simulink model "QCar_Workspace_studio"  (R2022b)
settings: Solver=ode1  StartTime=0.0  StopTime=inf  FixedStep=1/500  RelTol=1e-3  EnableMultiTasking=on
model workspace (MAT data in the model file):
  cameraStepSize = Simulink.Parameter
  cameraStepSize.Value = Simulink.data.Expression
  cameraStepSize.Value.ExpressionString = "qc_get_step_size * 2 + 0*ceil (1/90 /qc_get_step_size)"
  cameraStepSize.DataType = 'auto'
  cameraStepSize.Complexity = 'real'
  cameraStepSize.Dimensions = -1
  internalStepSize = Simulink.Parameter
  internalStepSize.Value = Simulink.data.Expression
  internalStepSize.Value.ExpressionString = "qc_get_step_size * ceil(1/120 /qc_get_step_size)"
  internalStepSize.DataType = 'auto'
  internalStepSize.Complexity = 'real'
  internalStepSize.Dimensions = -1
  mainStepSize = Simulink.Parameter
  mainStepSize.Value = Simulink.data.Expression
  mainStepSize.Value.ExpressionString = "qc_get_step_size"
  mainStepSize.DataType = 'auto'
  mainStepSize.Complexity = 'real'
  mainStepSize.Dimensions = -1
undefined symbols (not defined in the file or in its folder): qc_get_step_size
libraries: quarc_library x44, simulink x5
(part 1 of 2)
settings Model: SimulationMode=external  ExtModeTrigDuration=10000  Creator=mbohra  LastModifiedBy=mbohra
settings SolverCC: AlgebraicLoopSolver=TrustRegion  PositivePriorityOrder=on
settings DataIOCC: SaveOutput=off  SignalLogging=off  DSMLogging=off  SaveTime=off  ReturnWorkspaceOutputs=off
settings DebuggingCC: UnconnectedInputMsg=warning  UnconnectedOutputMsg=warning  UnconnectedLineMsg=warning  SFMachineParentedDataDiag=warning  ArithmeticOperatorsInVariantConditions=warning
settings ModelReferenceCC: EnableRefExpFcnMdlSchedulingChecks=on
settings SFSimCC: SimUseLocalCustomCode=off  CustomCodeUndefinedFunction=UseInterfaceOnly
settings RTWCC: Description=QUARC Win64 Target Using Toolchain  SystemTargetFile=quarc_win64.tlc  TemplateMakefile=quarc_default_tmf  RTWUseLocalCustomCode=off  Toolchain=QUARC win64 | nmake (64-bit Windows)  BuildConfiguration=Faster Runs  DLArmComputeVersion=19.05
settings CodeAppCC: StateflowObjectComments=on
settings STFCustomTargetCC: TargetLangStandard=C99 (ISO)  ConcurrentExecutionCompliant=on  GRTInterface=on  UseToolchainInfoCompliant=on  SystemTargetFile=quarc_win64.tlc
settings GRTTargetCC: ParMdlRefBuildCompliant=off  CompOptLevelCompliant=off  CombineOutputUpdateFcns=off  MatFileLogging=off  CPPClassGenCompliant=off  GRTInterface=on  ExtMode=on  ExtModeMexFile=quarc_comm
settings ConfigComp: CovMetricSettings=dswe

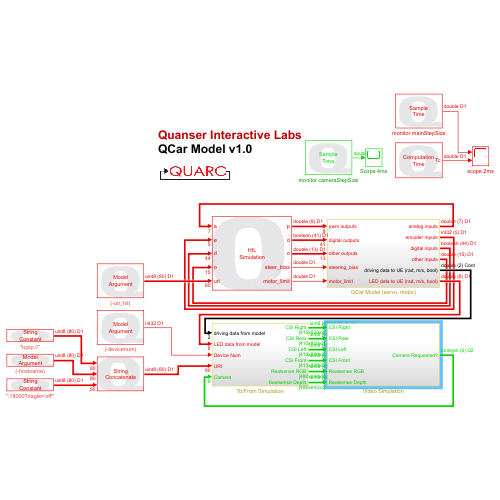
[thumbnail: Simulink's stored preview of the top-level diagram]
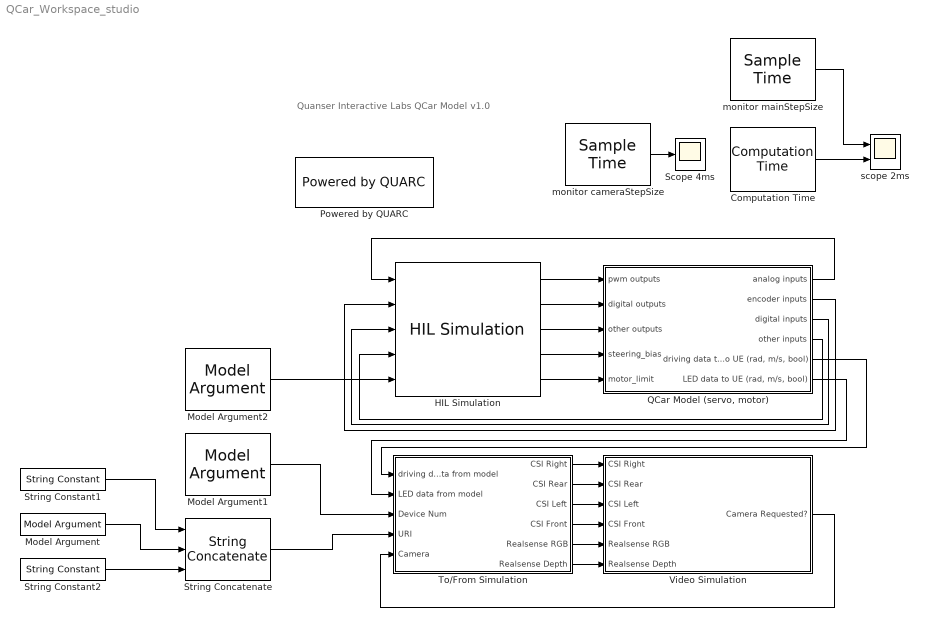
== system QCar_Workspace_studio ==
  note: Quanser Interactive Labs
      | QCar Model v1.0
  Computation Time : quarc_library/Sources/Time/Computation Time  sample_time=mainStepSize  use_model=on  use_cpu_time=off
  HIL Simulation : quarc_library/Data Acquisition/Generic/Configuration/HIL Simulation  uri_source=External input port  uri=tcpip://localhost:18960  board_type=qcar  board_id=0  options=steer_bias=%f;motor_limit=%f  sample_time=qc_get_step_size  active=on  num_clocks=1  num_interrupts=0  num_analog_inputs=7  num_analog_outputs=0  initial_analog=[]  num_digital_io=40  num_digital_inputs=4  num_digital_outputs=1  initial_digital=[]  num_encoder_inputs=5  num_pwm_outputs=8  initial_pwm=[]  other_inputs=[3000:3002, 4000:4002, 8000:8002, 10000, 14000:14004]  other_outputs=[1000, 11000:11011]  initial_other=[]  integer_get_property_codes=[]  double_get_property_codes=[]  string_get_property_codes=[]  integer_set_property_codes=[]  double_set_property_codes=[]  string_set_property_codes=[]  initial_integer_properties=0  initial_double_properties=0  initial_string_properties=[]  max_string_property=80  use_variable_size_strings=off
      settings: SourceProductName=QUARC Targets
  Model Argument : quarc_library/Sources/Signals/Model Argument  argument_name=hostname  has_value=on  data_type_mode=Specify via dialog  data_type=char  max_length=80  default_value=0  default_string=localhost  variable_size=off
      settings: AttributesFormatString=(-%<argument_name>)  SourceProductName=QUARC Targets
  Model Argument1 : quarc_library/Sources/Signals/Model Argument  argument_name=devicenum  has_value=on  data_type_mode=Specify via dialog  data_type=int32  max_length=80  default_value=0  variable_size=off
      settings: AttributesFormatString=(-%<argument_name>)  SourceProductName=QUARC Targets
  Model Argument2 : quarc_library/Sources/Signals/Model Argument  argument_name=uri_hil  has_value=on  data_type_mode=Specify via dialog  data_type=char  max_length=80  default_value=0  default_string=tcpip://localhost:18960  variable_size=off
      settings: AttributesFormatString=(-%<argument_name>)  SourceProductName=QUARC Targets
  Powered by QUARC : quarc_library/Logos/Powered by QUARC
  "QCar Model (servo, motor)" : Subsystem
  Scope 4ms : Scope
  String Concatenate : quarc_library/Strings/String Concatenate  num_inputs=3  max_length=80  output_size=Inherit from input
      settings: SourceProductName=QUARC Targets
  String Constant1 : quarc_library/Strings/String Constant  string_value=tcpip://  evaluate_string=off  string_type=text  max_length=80  sample_time=inf  variable_size=off
      settings: AttributesFormatString="\"tcpip://\""  SourceProductName=QUARC Targets
  String Constant2 : quarc_library/Strings/String Constant  string_value=:18000?nagle='off'  evaluate_string=off  string_type=text  max_length=80  sample_time=inf  variable_size=off
      settings: AttributesFormatString="\":18000?nagle='off'\""  SourceProductName=QUARC Targets
  To/From Simulation : Subsystem
  Video Simulation : Subsystem
  monitor cameraStepSize : quarc_library/Sources/Time/Sample Time  Priority=-99  sample_time=cameraStepSize
  monitor mainStepSize : quarc_library/Sources/Time/Sample Time  Priority=-99  sample_time=mainStepSize
  scope 2ms : Scope  NumInputPorts=2
  wires:
  To/From Simulation/1(CSI Right) -> Video Simulation/1(CSI Right)
  To/From Simulation/3(CSI Left) -> Video Simulation/3(CSI Left)
  To/From Simulation/5(Realsense RGB) -> Video Simulation/5(Realsense RGB)
  "QCar Model (servo, motor)"/5("driving data to UE (rad, m/s, bool)") -> To/From Simulation/1(driving data from model)
  To/From Simulation/2(CSI Rear) -> Video Simulation/2(CSI Rear)
  Model Argument1/1 -> To/From Simulation/3(Device Num)
  To/From Simulation/4(CSI Front) -> Video Simulation/4(CSI Front)
  HIL Simulation/5 -> "QCar Model (servo, motor)"/5(motor_limit)
  "QCar Model (servo, motor)"/6("LED data to UE (rad, m/s, bool)") -> To/From Simulation/2(LED data from model)
  To/From Simulation/6(Realsense Depth) -> Video Simulation/6(Realsense Depth)
  HIL Simulation/3 -> "QCar Model (servo, motor)"/3(other outputs)
  HIL Simulation/2 -> "QCar Model (servo, motor)"/2(digital outputs)
  "QCar Model (servo, motor)"/2(encoder inputs) -> HIL Simulation/2
  "QCar Model (servo, motor)"/3(digital inputs) -> HIL Simulation/3
  "QCar Model (servo, motor)"/1(analog inputs) -> HIL Simulation/1
  monitor cameraStepSize/1 -> Scope 4ms/1
  HIL Simulation/4 -> "QCar Model (servo, motor)"/4(steering_bias)
  monitor mainStepSize/1 -> scope 2ms/1
  "QCar Model (servo, motor)"/4(other inputs) -> HIL Simulation/4
  Video Simulation/1(Camera Requested?) -> To/From Simulation/5(Camera)
  HIL Simulation/1 -> "QCar Model (servo, motor)"/1(pwm outputs)
  Computation Time/1 -> scope 2ms/2
  String Constant1/1 -> String Concatenate/1
  Model Argument/1 -> String Concatenate/2
  String Constant2/1 -> String Concatenate/3
  String Concatenate/1 -> To/From Simulation/4(URI)
  Model Argument2/1 -> HIL Simulation/5

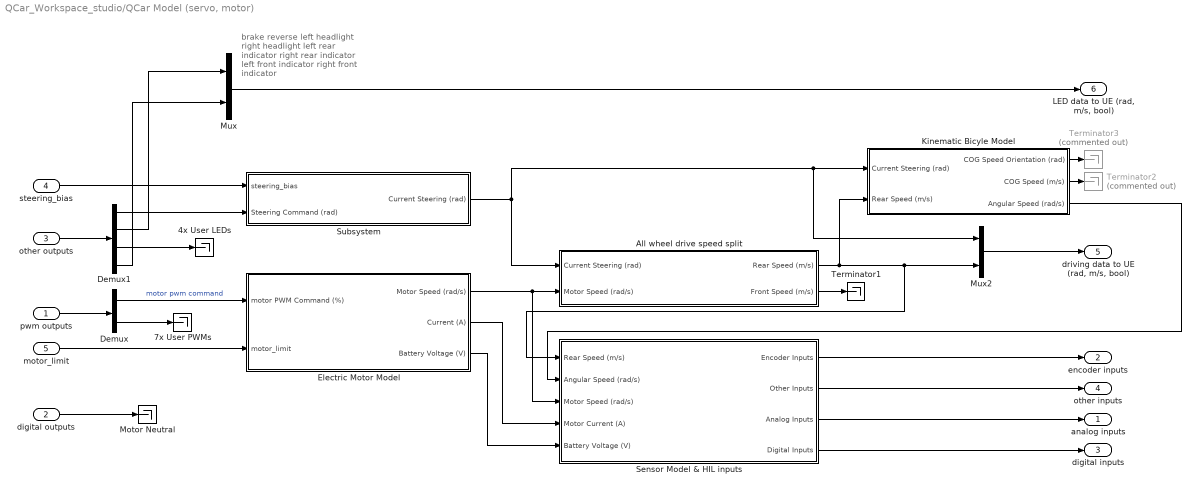
== system QCar_Workspace_studio/QCar Model (servo, motor) ==
  note: brake
      | reverse
      | left headlight
      | right headlight
      | left rear indicator
      | right rear indicator
      | left front indicator
      | right front indicator
  pwm outputs : Inport
  digital outputs : Inport  Port=2
  other outputs : Inport  Port=3
  steering_bias : Inport  Port=4
  motor_limit : Inport  Port=5
  4x User LEDs : Terminator
  7x User PWMs : Terminator
  All wheel drive speed split : Subsystem
  Demux : Demux  Outputs=[1 7]
  Demux1 : Demux  Outputs=[1 4 4 4]
  Electric Motor Model : Subsystem
  Kinematic Bicyle Model : Subsystem
  Motor Neutral : Terminator
  Mux : Mux  Inputs=2
  Mux2 : Mux  Inputs=2
  Sensor Model & HIL inputs : Subsystem
  Subsystem : Subsystem
  Terminator1 : Terminator
  Terminator2 : Terminator  Commented=on
  Terminator3 : Terminator  Commented=on
  analog inputs : Outport
  encoder inputs : Outport  Port=2  VectorParamsAs1DForOutWhenUnconnected=off
  digital inputs : Outport  Port=3
  other inputs : Outport  Port=4  VectorParamsAs1DForOutWhenUnconnected=off
  "driving data to UE (rad, m/s, bool)" : Outport  Port=5
  "LED data to UE (rad, m/s, bool)" : Outport  Port=6
  wires:
  Mux2/1 -> "driving data to UE (rad, m/s, bool)"/1
  All wheel drive speed split/1(Rear Speed (m/s)) -> Sensor Model & HIL inputs/1(Rear Speed (m/s)), Mux2/2, Kinematic Bicyle Model/2(Rear Speed (m/s))
  pwm outputs/1 -> Demux/1
  Electric Motor Model/1(Motor Speed (rad/s)) -> Sensor Model & HIL inputs/3(Motor Speed (rad/s)), All wheel drive speed split/2(Motor Speed (rad/s))
  Electric Motor Model/2(Current (A)) -> Sensor Model & HIL inputs/4(Motor Current (A))
  Electric Motor Model/3(Battery Voltage (V)) -> Sensor Model & HIL inputs/5(Battery Voltage (V))
  Sensor Model & HIL inputs/1(Encoder Inputs) -> encoder inputs/1
  Sensor Model & HIL inputs/2(Other Inputs) -> other inputs/1
  Sensor Model & HIL inputs/3(Analog Inputs) -> analog inputs/1
  All wheel drive speed split/2(Front Speed (m/s)) -> Terminator1/1
  Subsystem/1(Current Steering (rad)) -> Mux2/1, Kinematic Bicyle Model/1(Current Steering (rad)), All wheel drive speed split/1(Current Steering (rad))
  other outputs/1 -> Demux1/1
  Kinematic Bicyle Model/2(COG Speed (m/s)) -> Terminator2/1
  Kinematic Bicyle Model/1(COG Speed Orientation (rad)) -> Terminator3/1
  Demux/1 -> Electric Motor Model/1(motor PWM Command (%))  "motor pwm command"
  Demux/2 -> 7x User PWMs/1
  digital outputs/1 -> Motor Neutral/1
  Demux1/1 -> Subsystem/2(Steering Command (rad))
  Demux1/2 -> Mux/1
  Demux1/4 -> Mux/2
  Demux1/3 -> 4x User LEDs/1
  Mux/1 -> "LED data to UE (rad, m/s, bool)"/1
  Sensor Model & HIL inputs/4(Digital Inputs) -> digital inputs/1
  steering_bias/1 -> Subsystem/1(steering_bias)
  motor_limit/1 -> Electric Motor Model/2(motor_limit)
  Kinematic Bicyle Model/3(Angular Speed (rad/s)) -> Sensor Model & HIL inputs/2(Angular Speed (rad/s))

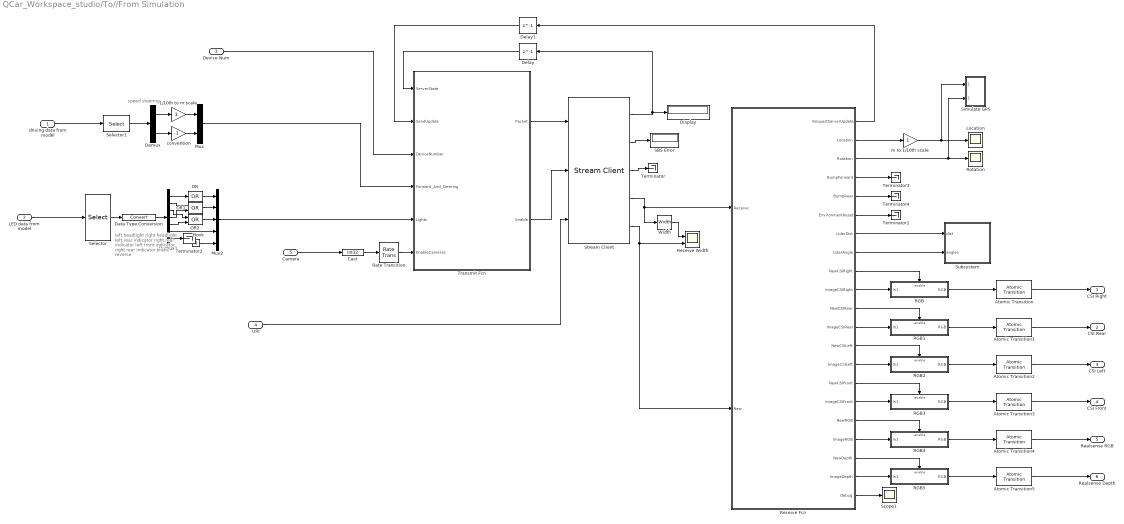
== system QCar_Workspace_studio/To//From Simulation ==
  note: speed
      | steering
  note: left headlight
      | right headlight
      | left rear indicator
      | right rear indicator
      | left front indicator
      | right rear indicator
      | brake
      | reverse
  driving data from model : Inport
  LED data from model : Inport  Port=2
  Device Num : Inport  Port=3
  URI : Inport  Port=4
  Camera : Inport  Port=5
  1/10th to m scale : Gain
  Atomic Transition{,1..5} (6 alike) : quarc_library/Advanced/Asynchronous/Atomic Transition  sample_time=cameraStepSize  data_type=Inherit: Same as input
      settings: SourceProductName=QUARC Targets
  Cast : DataTypeConversion  OutDataTypeStr=int32  SaturateOnIntegerOverflow=off  RndMeth=Floor
  Data Type Conversion : DataTypeConversion  SaturateOnIntegerOverflow=off  RndMeth=Floor
  Delay : Delay  DelayLength=1
  Delay1 : Delay  DelayLength=1
  Demux : Demux  Outputs=2
  Demux1 : Demux  Outputs=[2 1 1 1 1 1 1]
  Display : Display
  Honk : Constant  Value=0  OutDataTypeStr=boolean
  Location : Scope
  Mux : Mux  Inputs=2
  Mux2 : Mux  Inputs=5
  OR : Logic  Operator=OR  Inputs=1  IconShape=distinctive  AllPortsSameDT=off
  OR1 : Logic  Operator=OR  IconShape=distinctive  AllPortsSameDT=off  OutDataTypeStr=boolean
  OR2 : Logic  Operator=OR  IconShape=distinctive  AllPortsSameDT=off  OutDataTypeStr=boolean
  RGB : Subsystem
  RGB1 : Subsystem
  RGB2 : Subsystem
  RGB3 : Subsystem
  RGB4 : Subsystem
  RGB5 : Subsystem
  Rate Transition : RateTransition
  Receive Fcn : MATLAB Function  TreatAsAtomicUnit=on
  Receive Width : Scope  NumInputPorts=2
  Rotation : Scope
  SBS Error : Display
  Scope1 : Scope
  Selector : Selector  InputPortWidth=8  IndexOptions=Index vector (dialog)  Indices=[3 4 5 6 7 8 1 2 ]  OutputSizes=1
  Selector1 : Selector  InputPortWidth=2  IndexOptions=Index vector (dialog)  Indices=[2 1]  OutputSizes=1
  Simulate GPS : Subsystem
  Stream Client : quarc_library/Communications/Basic/Stream Client  uri_source=External input port  uri=tcpip://localhost:18000?nagle='off'  send_buffer_size=100000  receive_buffer_size=800000  byte_order=little endian (Intel - LSB first)  optimization=Minimum latency  send_options=Send all data  receive_options=Receive all data  default_value=[0]  sample_time=qc_get_step_size  active=on  implementation=Use blocking I/O in a separate thread  send_fifo_size=2  receive_fifo_size=2  send_priority=0  receive_priority=0  send_dimensions=on  receive_dimensions=on  max_dimensions=800000  data_type=uint8  type_expr=BusObject
  Subsystem : Subsystem
  Terminator{,1..4} (5 alike) : Terminator
  Transmit Fcn : MATLAB Function  TreatAsAtomicUnit=on
  Width : Width
  convention : Gain  Gain=-1
  m to 1/10th scale : Gain
  CSI Right : Outport
  CSI Rear : Outport  Port=2
  CSI Left : Outport  Port=3
  CSI Front : Outport  Port=4
  Realsense RGB : Outport  Port=5
  Realsense Depth : Outport  Port=6
  wires:
  Device Num/1 -> Transmit Fcn/3(DeviceNumber)
  LED data from model/1 -> Selector/1
  OR2/1 -> Mux2/3
  Demux1/7 -> Terminator2/1
  Selector/1 -> Data Type Conversion/1
  Demux1/4 -> OR1/2
  Data Type Conversion/1 -> Demux1/1
  Demux1/6 -> Mux2/4
  Demux1/3 -> OR2/1
  1/10th to m scale/1 -> Mux/1
  OR1/1 -> Mux2/2
  Selector1/1 -> Demux/1
  driving data from model/1 -> Selector1/1
  Demux1/5 -> OR2/2
  Honk/1 -> Mux2/5
  Demux/2 -> convention/1
  Demux1/1 -> OR/1
  OR/1 -> Mux2/1
  Demux1/2 -> OR1/1
  convention/1 -> Mux/2
  Demux/1 -> 1/10th to m scale/1
  Transmit Fcn/2(Enable) -> Stream Client/2
  Atomic Transition4/1 -> Realsense RGB/1
  Receive Fcn/10(ImageCSIRight) -> RGB/1(In1)
  RGB5/1(RGB) -> Atomic Transition5/1
  Width/1 -> Receive Width/1
  Receive Fcn/17(NewRGB) -> RGB4/Enable
  RGB3/1(RGB) -> Atomic Transition3/1
  Receive Fcn/13(NewCSILeft) -> RGB2/Enable
  Receive Fcn/12(ImageCSIRear) -> RGB1/1(In1)
  Receive Fcn/16(ImageCSIFront) -> RGB3/1(In1)
  Receive Fcn/9(NewCSIRight) -> RGB/Enable
  Receive Fcn/8(LidarAngle) -> Subsystem/2(angles)
  Receive Fcn/5(BumpRear) -> Terminator4/1
  RGB1/1(RGB) -> Atomic Transition1/1
  Atomic Transition5/1 -> Realsense Depth/1
  RGB4/1(RGB) -> Atomic Transition4/1
  Receive Fcn/1(RequestServerUpdate) -> Delay1/1
  Stream Client/2 -> SBS Error/1
  Atomic Transition2/1 -> CSI Left/1
  Receive Fcn/7(LidarDist) -> Subsystem/1(dist)
  Receive Fcn/20(ImageDepth) -> RGB5/1(In1)
  Receive Fcn/21(Debug) -> Scope1/1
  Receive Fcn/18(ImageRGB) -> RGB4/1(In1)
  RGB2/1(RGB) -> Atomic Transition2/1
  Atomic Transition3/1 -> CSI Front/1
  Stream Client/1 -> Display/1, Delay/1
  Stream Client/5 -> Receive Fcn/2(New), Receive Width/2
  Receive Fcn/15(NewCSIFront) -> RGB3/Enable
  Receive Fcn/19(NewDepth) -> RGB5/Enable
  Receive Fcn/14(ImageCSILeft) -> RGB2/1(In1)
  Delay/1 -> Transmit Fcn/1(ServerState)
  Receive Fcn/11(NewCSIRear) -> RGB1/Enable
  m to 1/10th scale/1 -> Simulate GPS/1(Position), Location/1
  Receive Fcn/3(Rotation) -> Simulate GPS/2(Rotation), Rotation/1
  RGB/1(RGB) -> Atomic Transition/1
  Atomic Transition1/1 -> CSI Rear/1
  Receive Fcn/2(Location) -> m to 1/10th scale/1
  Delay1/1 -> Transmit Fcn/2(SendUpdate)
  Cast/1 -> Rate Transition/1
  Receive Fcn/4(BumpForward) -> Terminator3/1
  Transmit Fcn/1(Packet) -> Stream Client/1
  Stream Client/4 -> Width/1, Receive Fcn/1(Receive)
  Stream Client/3 -> Terminator/1
  Mux/1 -> Transmit Fcn/4(Forward_And_Steering)
  Mux2/1 -> Transmit Fcn/5(Lights)
  Receive Fcn/6(EnvironmentReset) -> Terminator1/1
  Rate Transition/1 -> Transmit Fcn/6(EnableCameras)
  Atomic Transition/1 -> CSI Right/1
  URI/1 -> Stream Client/3
  Camera/1 -> Cast/1

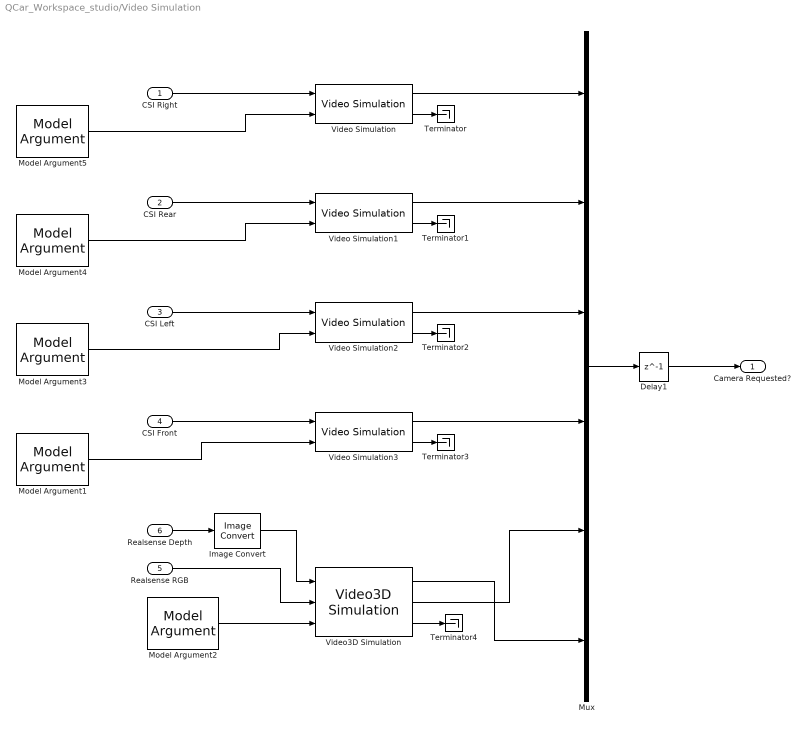
== system QCar_Workspace_studio/Video Simulation ==
  CSI Right : Inport
  CSI Rear : Inport  Port=2
  CSI Left : Inport  Port=3
  CSI Front : Inport  Port=4
  Realsense RGB : Inport  Port=5
  Realsense Depth : Inport  Port=6
  Delay1 : Delay  DelayLength=1  InitialCondition=[0 0 0 0 0 0]
  Image Convert : quarc_library/Image Processing/Generic/Image Convert  input_format=MATLAB RGB (HxWx3)  padding=0  output_format=MATLAB greyscale (HxW)  data_type=uint8
      settings: AttributesFormatString=(%<input_format>)  SourceProductName=QUARC Targets
  Model Argument1 : quarc_library/Sources/Signals/Model Argument  argument_name=uri_video3  has_value=on  data_type_mode=Specify via dialog  data_type=char  max_length=80  default_value=0  default_string=tcpip://localhost:18964  variable_size=off
      settings: AttributesFormatString=(-%<argument_name>)  SourceProductName=QUARC Targets
  Model Argument2 : quarc_library/Sources/Signals/Model Argument  argument_name=uri_video3d  has_value=on  data_type_mode=Specify via dialog  data_type=char  max_length=80  default_value=0  default_string=tcpip://localhost:18965  variable_size=off
      settings: AttributesFormatString=(-%<argument_name>)  SourceProductName=QUARC Targets
  Model Argument3 : quarc_library/Sources/Signals/Model Argument  argument_name=uri_video2  has_value=on  data_type_mode=Specify via dialog  data_type=char  max_length=80  default_value=0  default_string=tcpip://localhost:18963  variable_size=off
      settings: AttributesFormatString=(-%<argument_name>)  SourceProductName=QUARC Targets
  Model Argument4 : quarc_library/Sources/Signals/Model Argument  argument_name=uri_video1  has_value=on  data_type_mode=Specify via dialog  data_type=char  max_length=80  default_value=0  default_string=tcpip://localhost:18962  variable_size=off
      settings: AttributesFormatString=(-%<argument_name>)  SourceProductName=QUARC Targets
  Model Argument5 : quarc_library/Sources/Signals/Model Argument  argument_name=uri_video0  has_value=on  data_type_mode=Specify via dialog  data_type=char  max_length=80  default_value=0  default_string=tcpip://localhost:18961  variable_size=off
      settings: AttributesFormatString=(-%<argument_name>)  SourceProductName=QUARC Targets
  Mux : Mux  Inputs=6
  Terminator{,1..4} (5 alike) : Terminator
  Video Simulation : quarc_library/Multimedia/Video Simulation  uri_source=External input port  uri=tcpip://localhost:18961  device_id=0  widths=[820]  heights=[410]  rates=[30]  sample_time=cameraStepSize  show_in_use=on  active=on
      settings: SourceProductName=QUARC Targets
  Video Simulation1 : quarc_library/Multimedia/Video Simulation  uri_source=External input port  uri=tcpip://localhost:18962  device_id=1  widths=[820]  heights=[410]  rates=[30]  sample_time=cameraStepSize  show_in_use=on  active=on
      settings: SourceProductName=QUARC Targets
  Video Simulation2 : quarc_library/Multimedia/Video Simulation  uri_source=External input port  uri=tcpip://localhost:18963  device_id=2  widths=[820]  heights=[410]  rates=[30]  sample_time=cameraStepSize  show_in_use=on  active=on
      settings: SourceProductName=QUARC Targets
  Video Simulation3 : quarc_library/Multimedia/Video Simulation  uri_source=External input port  uri=tcpip://localhost:18964  device_id=3  widths=[820]  heights=[410]  rates=[30]  sample_time=cameraStepSize  show_in_use=on  active=on
      settings: SourceProductName=QUARC Targets
  Video3D Simulation : quarc_library/Multimedia/Video3D Simulation  uri_source=External input port  uri=tcpip://localhost:18965  device_id=0  sample_time=cameraStepSize  show_in_use=on  active=on  depth_indices=[0]  depth_scales=9.44  depth_widths=[640]  depth_heights=[480]  depth_rates=[30]  rgb_indices=[0]  rgb_widths=[640]  rgb_heights=[480]  rgb_rates=[30]  infrared_indices=[]  infrared_widths=[640]  infrared_heights=[480]  infrared_rates=[90]  fisheye_indices=[]  fisheye_widths=[640]  fisheye_heights=[480]  fisheye_rates=[30]  gyro_indices=[]  accel_indices=[]  pose_indices=[]
      settings: SourceProductName=QUARC Targets
  Camera Requested? : Outport
  wires:
  Video3D Simulation/1 -> Mux/6
  Video3D Simulation/2 -> Mux/5
  Video3D Simulation/3 -> Terminator4/1
  Video Simulation/1 -> Mux/1
  Video Simulation3/2 -> Terminator3/1
  Video Simulation1/1 -> Mux/2
  Video Simulation2/2 -> Terminator2/1
  CSI Right/1 -> Video Simulation/1
  Video Simulation2/1 -> Mux/3
  Video Simulation3/1 -> Mux/4
  Video Simulation1/2 -> Terminator1/1
  Video Simulation/2 -> Terminator/1
  Realsense RGB/1 -> Video3D Simulation/2
  CSI Rear/1 -> Video Simulation1/1
  CSI Left/1 -> Video Simulation2/1
  Realsense Depth/1 -> Image Convert/1
  Mux/1 -> Delay1/1
  Delay1/1 -> Camera Requested?/1
  Image Convert/1 -> Video3D Simulation/1
  CSI Front/1 -> Video Simulation3/1
  Model Argument2/1 -> Video3D Simulation/3
  Model Argument1/1 -> Video Simulation3/2
  Model Argument3/1 -> Video Simulation2/2
  Model Argument4/1 -> Video Simulation1/2
  Model Argument5/1 -> Video Simulation/2

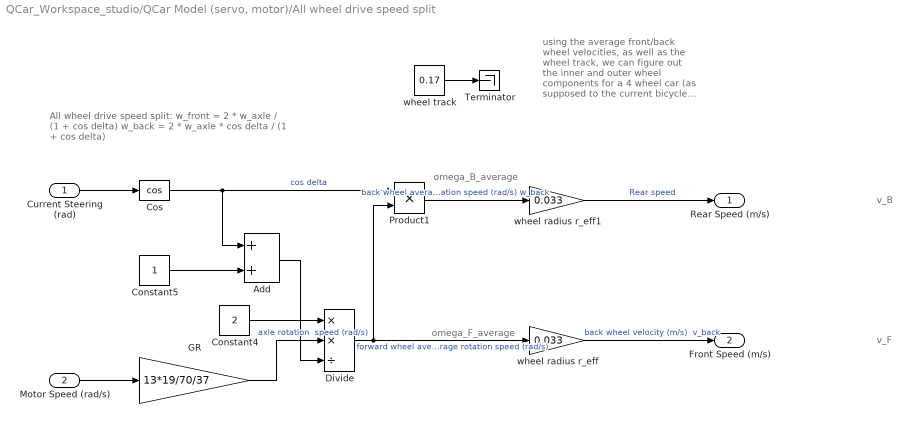
== system QCar_Workspace_studio/QCar Model (servo, motor)/All wheel drive speed split ==
  note: v_B
  note: All wheel drive speed split:
      | w_front = 2 * w_axle / (1 + cos delta)
      | w_back = 2 * w_axle * cos delta / (1 + cos delta)
  note: using the average front/back
      | wheel velocities, as well as the
      | wheel track, we can figure out
      | the inner and outer wheel
      | components for a 4 wheel
      | car (as supposed to the current
      | bicycle model).
  note: v_F
  note: omega_B_average
  note: omega_F_average
  Current Steering (rad) : Inport
  Motor Speed (rad/s) : Inport  Port=2
  Add : Sum
  Constant4 : Constant  Value=2
  Constant5 : Constant
  Cos : Trigonometry  Operator=cos
  Divide : Product  Inputs=**/
  GR : Gain  Gain=13*19/70/37
  Product1 : Product
  Terminator : Terminator
  wheel radius r_eff : Gain  Gain=0.033
  wheel radius r_eff1 : Gain  Gain=0.033
  wheel track : Constant  Value=0.17
  Rear Speed (m/s) : Outport
  Front Speed (m/s) : Outport  Port=2
  wires:
  GR/1 -> Divide/2  "axle rotation  speed (rad/s)"
  Cos/1 -> Add/1, Product1/1  "cos delta"
  Divide/1 -> wheel radius r_eff/1, Product1/2  "forward wheel average rotation speed (rad/s)"
  Constant5/1 -> Add/2
  Add/1 -> Divide/3
  Constant4/1 -> Divide/1
  Motor Speed (rad/s)/1 -> GR/1
  Current Steering (rad)/1 -> Cos/1
  Product1/1 -> wheel radius r_eff1/1  "back wheel average rotation speed (rad/s) w_back"
  wheel track/1 -> Terminator/1
  wheel radius r_eff/1 -> Front Speed (m/s)/1  "back wheel velocity (m/s)  v_back"
  wheel radius r_eff1/1 -> Rear Speed (m/s)/1  "Rear speed"

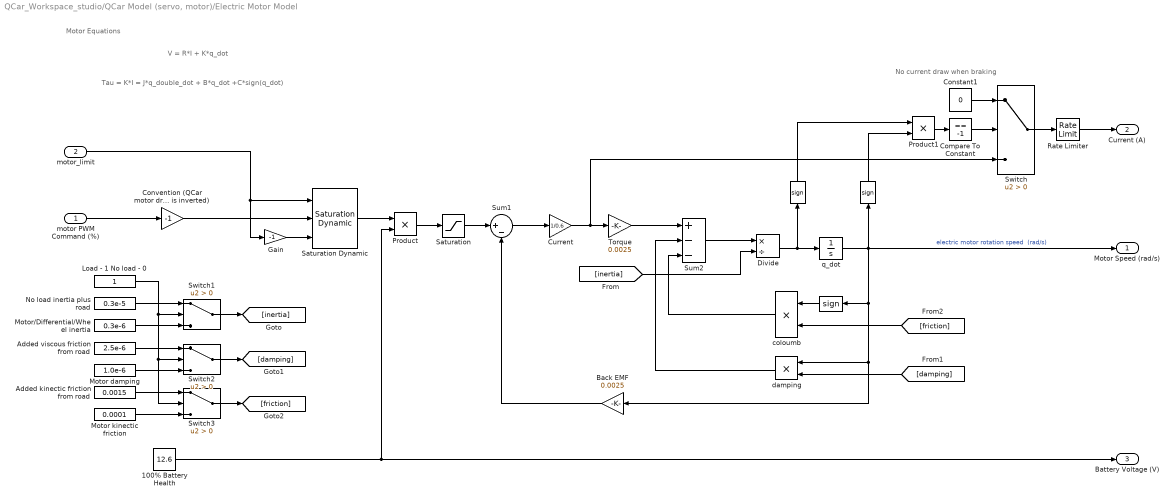
== system QCar_Workspace_studio/QCar Model (servo, motor)/Electric Motor Model ==
  note: No current draw when braking
  note: Motor Equations
  note: Tau = K*I = J*q_double_dot + B*q_dot +C*sign(q_dot)
  note: V = R*I + K*q_dot
  motor PWM Command (%) : Inport
  motor_limit : Inport  Port=2
  " " : Signum
  "  " : Signum
  "   " : Signum
  100% Battery Health : Constant  Value=12.6
  Added kinectic friction from road : Constant  Value=0.0015
  Added viscous friction from road : Constant  Value=2.5e-6
  Back EMF : Gain  Gain=0.0025
  Compare To Constant : simulink/Logic and Bit Operations/Compare To Constant  relop===  const=-1  OutDataTypeStr=boolean
  Constant1 : Constant  Value=0
  Convention (QCar motor drive is inverted) : Gain  Gain=-1
  Current : Gain  Gain=1/0.6
  Divide : Product  Inputs=*/
  Gain : Gain  Gain=-1
  Load - 1 No load - 0 : Constant
  Motor damping : Constant  Value=1.0e-6
  Motor kinectic friction : Constant  Value=0.0001
  Motor/Differential/Wheel inertia : Constant  Value=0.3e-6
  No load inertia plus road : Constant  Value=0.3e-5
  Product : Product
  Product1 : Product
  Rate Limiter : RateLimiter  RisingSlewLimit=1*10  FallingSlewLimit=-1*10  SampleTimeMode=inherited
  Saturation : Saturate  UpperLimit=12.6  LowerLimit=-12.6
  Saturation Dynamic : simulink/Discontinuities/Saturation Dynamic  OutMin=[]  OutMax=[]  OutDataTypeStr=Inherit: Same as second input  OutDataType=fixdt(1, 16)  OutScaling=2^-10  DoSatur=off
  Sum1 : Sum  Inputs=|+-
  Sum2 : Sum  Inputs=+--
  Switch{,1..3} (4 alike) : Switch  Criteria=u2 > Threshold  SaturateOnIntegerOverflow=off  InputSameDT=off
  Torque : Gain  Gain=0.0025
  coloumb : Product
  damping : Product
  q_dot : Integrator
  Motor Speed (rad/s) : Outport
  Current (A) : Outport  Port=2
  Battery Voltage (V) : Outport  Port=3
  wires:
  Back EMF/1 -> Sum1/2
  q_dot/1 -> "  "/1, " "/1, Back EMF/1, damping/1, Motor Speed (rad/s)/1  "electric motor rotation speed  (rad/s)"
  coloumb/1 -> Sum2/3
  Sum1/1 -> Current/1
  100% Battery Health/1 -> Product/2, Battery Voltage (V)/1
  Sum2/1 -> Divide/1
  Torque/1 -> Sum2/1
  "  "/1 -> Product1/2
  damping/1 -> Sum2/2
  Divide/1 -> q_dot/1, "   "/1
  Product/1 -> Saturation/1
  motor PWM Command (%)/1 -> Convention (QCar motor drive is inverted)/1
  Saturation Dynamic/1 -> Product/1
  motor_limit/1 -> Gain/1, Saturation Dynamic/1
  Gain/1 -> Saturation Dynamic/3
  Convention (QCar motor drive is inverted)/1 -> Saturation Dynamic/2
  [damping] -> damping/2
  [friction] -> coloumb/2
  Current/1 -> Torque/1, Switch/3
  Saturation/1 -> Sum1/1
  "   "/1 -> Product1/1
  Product1/1 -> Compare To Constant/1
  Compare To Constant/1 -> Switch/2
  Constant1/1 -> Switch/1
  Switch/1 -> Rate Limiter/1
  Rate Limiter/1 -> Current (A)/1
  Load - 1 No load - 0/1 -> Switch2/2, Switch3/2, Switch1/2
  No load inertia plus road/1 -> Switch1/1
  Motor/Differential/Wheel inertia/1 -> Switch1/3
  Added viscous friction from road/1 -> Switch2/1
  Motor damping/1 -> Switch2/3
  Added kinectic friction from road/1 -> Switch3/1
  Motor kinectic friction/1 -> Switch3/3
  Switch1/1 -> [inertia]
  Switch2/1 -> [damping]
  Switch3/1 -> [friction]
  [inertia] -> Divide/2
  " "/1 -> coloumb/1

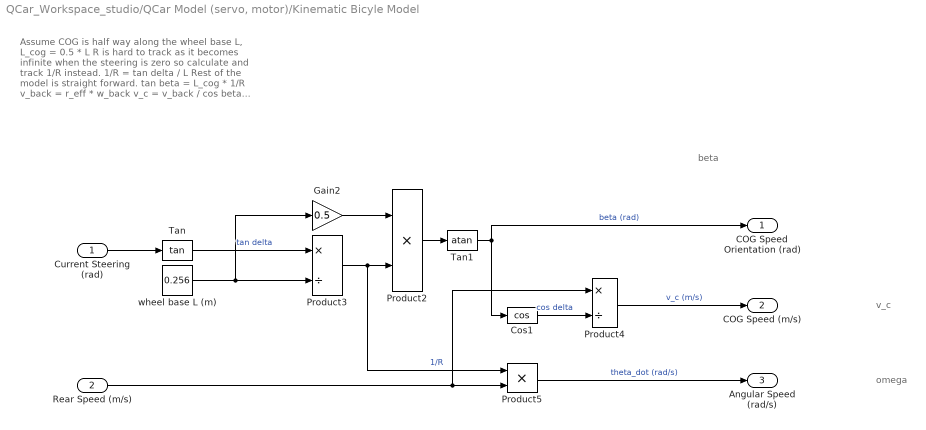
== system QCar_Workspace_studio/QCar Model (servo, motor)/Kinematic Bicyle Model ==
  note: beta
  note: Assume COG is half way along the wheel base L,
      | L_cog = 0.5 * L
      |
      | R is hard to track as it becomes infinite when
      | the steering is zero so calculate and track 1/R
      | instead.
      | 1/R = tan delta / L
      |
      | Rest of the model is straight forward.
      | tan beta = L_cog * 1/R
      | v_back = r_eff * w_back
      | v_c = v_back / cos beta
      | theta_dot = v_back * 1/R
  note: v_c
  note: omega
  Current Steering (rad) : Inport
  Rear Speed (m/s) : Inport  Port=2
  Cos1 : Trigonometry  Operator=cos
  Gain2 : Gain  Gain=0.5
  Product2 : Product
  Product3 : Product  Inputs=*/
  Product4 : Product  Inputs=*/
  Product5 : Product
  Tan : Trigonometry  Operator=tan
  Tan1 : Trigonometry  Operator=atan
  wheel base L (m) : Constant  Value=0.256
  COG Speed Orientation (rad) : Outport
  COG Speed (m/s) : Outport  Port=2
  Angular Speed (rad/s) : Outport  Port=3
  wires:
  Gain2/1 -> Product2/1
  wheel base L (m)/1 -> Gain2/1, Product3/2
  Product3/1 -> Product5/1, Product2/2  "1/R"
  Product2/1 -> Tan1/1
  Rear Speed (m/s)/1 -> Product4/1, Product5/2
  Cos1/1 -> Product4/2  "cos delta"
  Tan/1 -> Product3/1  "tan delta"
  Current Steering (rad)/1 -> Tan/1
  Product4/1 -> COG Speed (m/s)/1  "v_c (m/s)"
  Product5/1 -> Angular Speed (rad/s)/1  "theta_dot (rad/s)"
  Tan1/1 -> Cos1/1, COG Speed Orientation (rad)/1  "beta (rad)"

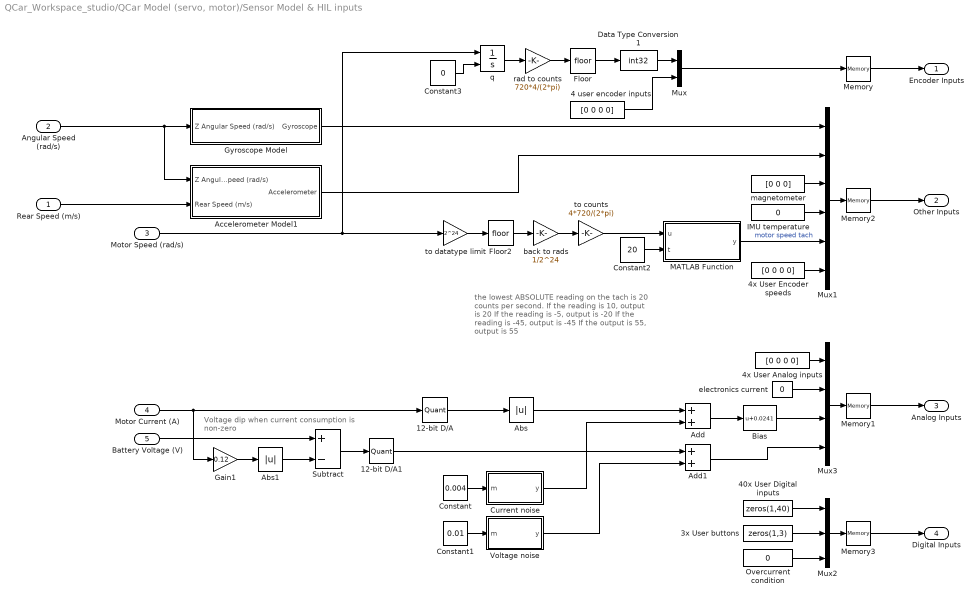
== system QCar_Workspace_studio/QCar Model (servo, motor)/Sensor Model & HIL inputs ==
  note: Voltage dip when current
      | consumption is non-zero
  note: the lowest ABSOLUTE reading on the tach
      | is 20 counts per second.
      |
      | If the reading is 10, output is 20
      | If the reading is -5, output is -20
      | If the reading is -45, output is -45
      | If the output is 55, output is 55
  Rear Speed (m/s) : Inport
  Angular Speed (rad/s) : Inport  Port=2
  Motor Speed (rad/s) : Inport  Port=3
  Motor Current (A) : Inport  Port=4
  Battery Voltage (V) : Inport  Port=5
  12-bit D/A : Quantizer  QuantizationInterval=1/2^12
  12-bit D/A1 : Quantizer  QuantizationInterval=1/2^12
  3x User buttons : Constant  Value=zeros(1,3)  OutDataTypeStr=boolean
  4 user encoder inputs : Constant  Value=[0 0 0 0]  OutDataTypeStr=int32
  40x User Digital inputs : Constant  Value=zeros(1,40)  OutDataTypeStr=boolean
  4x User Analog inputs : Constant  Value=[0 0 0 0]
  4x User Encoder speeds : Constant  Value=[0 0 0 0]
  Abs : Abs  SaturateOnIntegerOverflow=off
  Abs1 : Abs  SaturateOnIntegerOverflow=off
  Accelerometer Model1 : Subsystem
  Add : Sum
  Add1 : Sum
  Bias : Bias  Bias=0.0241  SaturateOnIntegerOverflow=off
  Constant : Constant  Value=0.004
  Constant1 : Constant  Value=0.01
  Constant2 : Constant  Value=20
  Constant3 : Constant  Value=0
  Current noise : MATLAB Function  TreatAsAtomicUnit=on
  Data Type Conversion1 : DataTypeConversion  OutDataTypeStr=int32  SaturateOnIntegerOverflow=off  RndMeth=Floor
  Floor : Rounding
  Floor2 : Rounding
  Gain1 : Gain  Gain=0.12
  Gyroscope Model : Subsystem
  IMU temperature : Constant  Value=0
  MATLAB Function : MATLAB Function  TreatAsAtomicUnit=on
  Memory : Memory  InitialCondition=[0 0 0 0 0]  InheritSampleTime=on
  Memory1 : Memory  InitialCondition=zeros(1, 7)
  Memory2 : Memory  InitialCondition=zeros(1, 15)
  Memory3 : Memory  InitialCondition=zeros(1,44)
  Mux : Mux  Inputs=2
  Mux1 : Mux  Inputs=6
  Mux2 : Mux  Inputs=3
  Mux3 : Mux
  Overcurrent condition : Constant  Value=0  OutDataTypeStr=boolean
  Subtract : Sum  Inputs=+-
  Voltage noise : MATLAB Function  TreatAsAtomicUnit=on
  back to rads : Gain  Gain=1/2^24
  electronics current : Constant  Value=0
  magnetometer : Constant  Value=[0 0 0]
  q : Integrator  ExternalReset=either
  rad to counts : Gain  Gain=720*4/(2*pi)
  to counts : Gain  Gain=4*720/(2*pi)
  to datatype limit : Gain  Gain=2^24
  Encoder Inputs : Outport
  Other Inputs : Outport  Port=2
  Analog Inputs : Outport  Port=3
  Digital Inputs : Outport  Port=4
  wires:
  Data Type Conversion1/1 -> Mux/1
  Mux1/1 -> Memory2/1
  4x User Analog inputs/1 -> Mux3/1
  Accelerometer Model1/1(Accelerometer) -> Mux1/2
  4x User Encoder speeds/1 -> Mux1/6
  electronics current/1 -> Mux3/2
  Mux3/1 -> Memory1/1
  Memory1/1 -> Analog Inputs/1
  Floor2/1 -> back to rads/1
  Memory/1 -> Encoder Inputs/1
  to counts/1 -> MATLAB Function/1(u)
  MATLAB Function/1(y) -> Mux1/5  "motor speed tach"
  Constant2/1 -> MATLAB Function/2(t)
  Add/1 -> Bias/1
  back to rads/1 -> to counts/1
  to datatype limit/1 -> Floor2/1
  IMU temperature/1 -> Mux1/4
  Motor Speed (rad/s)/1 -> q/1, to datatype limit/1
  Constant3/1 -> q/2
  Mux/1 -> Memory/1
  q/1 -> rad to counts/1
  Memory2/1 -> Other Inputs/1
  rad to counts/1 -> Floor/1
  magnetometer/1 -> Mux1/3
  Floor/1 -> Data Type Conversion1/1
  4 user encoder inputs/1 -> Mux/2
  Motor Current (A)/1 -> 12-bit D/A/1, Gain1/1
  40x User Digital inputs/1 -> Mux2/1
  Memory3/1 -> Digital Inputs/1
  Overcurrent condition/1 -> Mux2/3
  3x User buttons/1 -> Mux2/2
  Mux2/1 -> Memory3/1
  12-bit D/A/1 -> Abs/1
  Current noise/1(y) -> Add/2
  Abs/1 -> Add/1
  Bias/1 -> Mux3/3
  Constant/1 -> Current noise/1(m)
  Constant1/1 -> Voltage noise/1(m)
  Add1/1 -> Mux3/4
  Voltage noise/1(y) -> Add1/2
  12-bit D/A1/1 -> Add1/1
  Battery Voltage (V)/1 -> Subtract/1
  Gain1/1 -> Abs1/1
  Subtract/1 -> 12-bit D/A1/1
  Abs1/1 -> Subtract/2
  Angular Speed (rad/s)/1 -> Accelerometer Model1/1(Z Angular Speed (rad/s)), Gyroscope Model/1(Z Angular Speed (rad/s))
  Gyroscope Model/1(Gyroscope) -> Mux1/1
  Rear Speed (m/s)/1 -> Accelerometer Model1/2(Rear Speed (m/s))

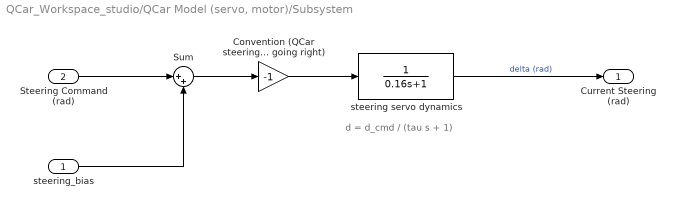
== system QCar_Workspace_studio/QCar Model (servo, motor)/Subsystem ==
  note: d = d_cmd / (tau s + 1)
  steering_bias : Inport
  Steering Command (rad) : Inport  Port=2
  Convention (QCar steering is +ve going right) : Gain  Gain=-1
  Sum : Sum  Inputs=|++
  steering servo dynamics : TransferFcn  Denominator=[0.16 1]
  Current Steering (rad) : Outport
  wires:
  steering servo dynamics/1 -> Current Steering (rad)/1  "delta (rad)"
  steering_bias/1 -> Sum/2
  Sum/1 -> Convention (QCar steering is +ve going right)/1
  Steering Command (rad)/1 -> Sum/1
  Convention (QCar steering is +ve going right)/1 -> steering servo dynamics/1

== system QCar_Workspace_studio/To//From Simulation/RGB ==
  In1 : Inport
  Enable : EnablePort  StatesWhenEnabling=reset
  Image Decompress : quarc_library/Image Processing/Generic/Image Decompress  algorithm=JPEG  resolution=custom  width=820  height=410  output_format=MATLAB RGB (HxWx3)  data_type=uint8
      settings: AttributesFormatString=(%<algorithm>)  SourceProductName=QUARC Targets
  RGB : Outport  VectorParamsAs1DForOutWhenUnconnected=off
  wires:
  In1/1 -> Image Decompress/1
  Image Decompress/1 -> RGB/1

== system QCar_Workspace_studio/To//From Simulation/RGB1 ==
  In1 : Inport
  Enable : EnablePort  StatesWhenEnabling=reset
  Image Decompress : quarc_library/Image Processing/Generic/Image Decompress  algorithm=JPEG  resolution=custom  width=820  height=410  output_format=MATLAB RGB (HxWx3)  data_type=uint8
      settings: AttributesFormatString=(%<algorithm>)  SourceProductName=QUARC Targets
  RGB : Outport  VectorParamsAs1DForOutWhenUnconnected=off
  wires:
  In1/1 -> Image Decompress/1
  Image Decompress/1 -> RGB/1

== system QCar_Workspace_studio/To//From Simulation/RGB2 ==
  In1 : Inport
  Enable : EnablePort  StatesWhenEnabling=reset
  Image Decompress : quarc_library/Image Processing/Generic/Image Decompress  algorithm=JPEG  resolution=custom  width=820  height=410  output_format=MATLAB RGB (HxWx3)  data_type=uint8
      settings: AttributesFormatString=(%<algorithm>)  SourceProductName=QUARC Targets
  RGB : Outport  VectorParamsAs1DForOutWhenUnconnected=off
  wires:
  In1/1 -> Image Decompress/1
  Image Decompress/1 -> RGB/1

== system QCar_Workspace_studio/To//From Simulation/RGB3 ==
  In1 : Inport
  Enable : EnablePort  StatesWhenEnabling=reset
  Image Decompress : quarc_library/Image Processing/Generic/Image Decompress  algorithm=JPEG  resolution=custom  width=820  height=410  output_format=MATLAB RGB (HxWx3)  data_type=uint8
      settings: AttributesFormatString=(%<algorithm>)  SourceProductName=QUARC Targets
  RGB : Outport  VectorParamsAs1DForOutWhenUnconnected=off
  wires:
  In1/1 -> Image Decompress/1
  Image Decompress/1 -> RGB/1

== system QCar_Workspace_studio/To//From Simulation/RGB4 ==
  In1 : Inport
  Enable : EnablePort  StatesWhenEnabling=reset
  Image Decompress : quarc_library/Image Processing/Generic/Image Decompress  algorithm=JPEG  resolution=640 x 480  width=640  height=480  output_format=MATLAB RGB (HxWx3)  data_type=uint8
      settings: AttributesFormatString=(%<algorithm>)  SourceProductName=QUARC Targets
  RGB : Outport  VectorParamsAs1DForOutWhenUnconnected=off
  wires:
  In1/1 -> Image Decompress/1
  Image Decompress/1 -> RGB/1

== system QCar_Workspace_studio/To//From Simulation/RGB5 ==
  In1 : Inport
  Enable : EnablePort  StatesWhenEnabling=reset
  Image Decompress : quarc_library/Image Processing/Generic/Image Decompress  algorithm=JPEG  resolution=640 x 480  width=640  height=480  output_format=MATLAB RGB (HxWx3)  data_type=uint8
      settings: AttributesFormatString=(%<algorithm>)  SourceProductName=QUARC Targets
  RGB : Outport  VectorParamsAs1DForOutWhenUnconnected=off
  wires:
  In1/1 -> Image Decompress/1
  Image Decompress/1 -> RGB/1

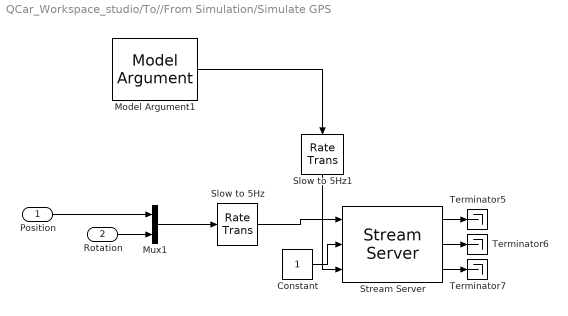
== system QCar_Workspace_studio/To//From Simulation/Simulate GPS ==
  Position : Inport
  Rotation : Inport  Port=2
  Constant : Constant
  Model Argument1 : quarc_library/Sources/Signals/Model Argument  argument_name=uri_gps  has_value=on  data_type_mode=Specify via dialog  data_type=char  max_length=80  default_value=0  default_string=tcpip://remotehost:18967  variable_size=off
      settings: AttributesFormatString=(-%<argument_name>)  SourceProductName=QUARC Targets
  Mux1 : Mux  Inputs=2
  Slow to 5Hz : RateTransition  OutPortSampleTime=qc_get_step_size*100
  Slow to 5Hz1 : RateTransition  OutPortSampleTime=qc_get_step_size*100
  Stream Server : quarc_library/Communications/Basic/Stream Server  uri_source=External input port  uri=tcpip://remotehost:18967  send_buffer_size=1460  receive_buffer_size=1460  byte_order=little endian (Intel - LSB first)  optimization=Minimum latency  send_options=Send most recent data  receive_options=Do not receive data  default_value=[0]  sample_time=qc_get_step_size*100  active=off  implementation=Use blocking I/O in a separate thread  send_fifo_size=1000  receive_fifo_size=1000  send_priority=0  receive_priority=0  send_dimensions=off  receive_dimensions=off  max_dimensions=-1  data_type=Inherited via back propagation  type_expr=BusObject
  Terminator5 : Terminator
  Terminator6 : Terminator
  Terminator7 : Terminator
  wires:
  Rotation/1 -> Mux1/2
  Stream Server/1 -> Terminator5/1
  Stream Server/2 -> Terminator6/1
  Stream Server/3 -> Terminator7/1
  Constant/1 -> Stream Server/2
  Position/1 -> Mux1/1
  Mux1/1 -> Slow to 5Hz/1
  Slow to 5Hz/1 -> Stream Server/1
  Model Argument1/1 -> Slow to 5Hz1/1
  Slow to 5Hz1/1 -> Stream Server/3

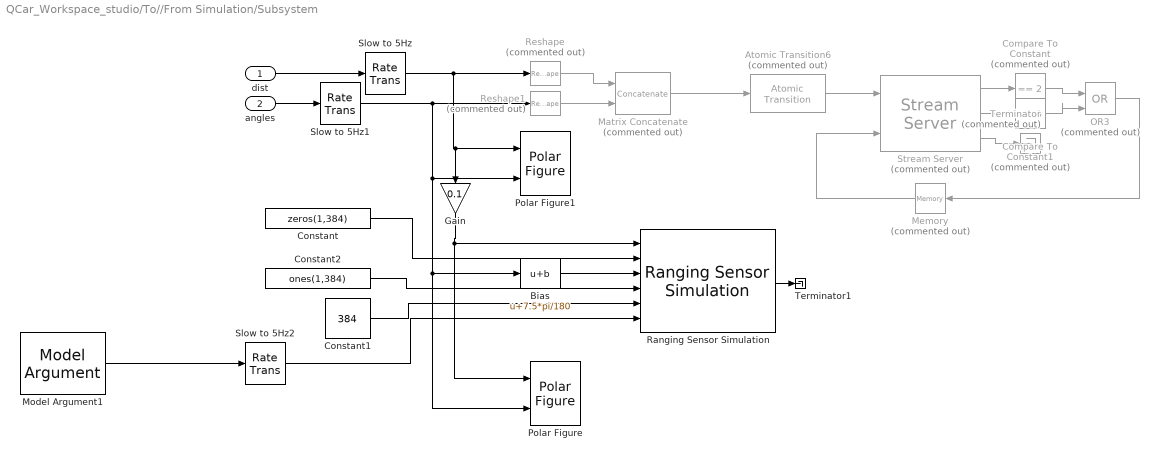
== system QCar_Workspace_studio/To//From Simulation/Subsystem ==
  dist : Inport
  angles : Inport  Port=2
  Atomic Transition6 : quarc_library/Advanced/Asynchronous/Atomic Transition  Commented=on  sample_time=cameraStepSize  data_type=Inherit: Same as input
      settings: SourceProductName=QUARC Targets
  Bias : Bias  Bias=7.5*pi/180  SaturateOnIntegerOverflow=off
  Compare To Constant : simulink/Logic and Bit Operations/Compare To Constant  Commented=on  relop===  const=2  OutDataTypeStr=boolean
  Compare To Constant1 : simulink/Logic and Bit Operations/Compare To Constant  Commented=on  relop=>=  const=0  OutDataTypeStr=boolean
  Constant : Constant  Value=zeros(1,384)
  Constant1 : Constant  Value=384
  Constant2 : Constant  Value=ones(1,384)
  Gain : Gain  Gain=0.1
  Matrix Concatenate : Concatenate  Commented=on  Mode=Multidimensional array  ConcatenateDimension=3
  Memory : Memory  Commented=on  InheritSampleTime=on
  Model Argument1 : quarc_library/Sources/Signals/Model Argument  argument_name=uri_lidar  has_value=on  data_type_mode=Specify via dialog  data_type=char  max_length=80  default_value=0  default_string=tcpip://localhost:18966  variable_size=off
      settings: AttributesFormatString=(-%<argument_name>)  SourceProductName=QUARC Targets
  OR3 : Logic  Commented=on  Operator=OR  IconShape=distinctive  AllPortsSameDT=off  OutDataTypeStr=boolean
  Polar Figure : quarc_library/Sinks/Figures/Polar Figure  figure_mode=Use figure window  figure_tag=figure1  axes_tag=axes1  plot_mode=Frame-based  minimum_rho=0  maximum_rho=2  minimum_theta=0  maximum_theta=360  zero_location=top  direction=counterclockwise  buffer_size=1  update_rate=100  sample_time=-1  initial_position="2   50  958  457"  initial_visibility=off  line1_style=Solid line (-)  line1_width=0.5  line1_color=[0 0.4470 0.7410]  marker1=Circle (o)  marker1_size=2  marker1_edge_color=[0 0.447059 0.741176]  marker1_face_color=[0 0.447059 0.741176]  line2_style=Solid line (-)  line2_width=0.5  line2_color=[0.85098 0.32549 0.0980392]  marker2=None  marker2_size=6  marker2_edge_color=[0.85098 0.32549 0.0980392]  marker2_face_color=[0.85098 0.32549 0.0980392]  line3_style=Solid line (-)  line3_width=0.5  line3_color=[0.929412 0.694118 0.12549]  marker3=None  marker3_size=6  marker3_edge_color=[0.929412 0.694118 0.12549]  marker3_face_color=[0.929412 0.694118 0.12549]  line4_style=Solid line (-)  line4_width=0.5  line4_color=[0.494118 0.184314 0.556863]  marker4=None  marker4_size=6  marker4_edge_color=[0.494118 0.184314 0.556863]  marker4_face_color=[0.494118 0.184314 0.556863]  line5_style=Solid line (-)  line5_width=0.5  line5_color=[0.466667 0.67451 0.188235]  marker5=None  marker5_size=6  marker5_edge_color=[0.466667 0.67451 0.188235]  marker5_face_color=[0.466667 0.67451 0.188235]
      settings: SourceProductName=QUARC Targets
  Polar Figure1 : quarc_library/Sinks/Figures/Polar Figure  figure_mode=Use figure window  figure_tag=figure1  axes_tag=axes1  plot_mode=Frame-based  minimum_rho=0  maximum_rho=80  minimum_theta=0  maximum_theta=360  zero_location=top  direction=clockwise  buffer_size=1  update_rate=100  sample_time=-1  initial_position="-3  566  963  457"  initial_visibility=off  line1_style=Solid line (-)  line1_width=0.5  line1_color=[0 0.4470 0.7410]  marker1=Circle (o)  marker1_size=2  marker1_edge_color=[0 0.447059 0.741176]  marker1_face_color=[0 0.447059 0.741176]  line2_style=Solid line (-)  line2_width=0.5  line2_color=[0.85098 0.32549 0.0980392]  marker2=None  marker2_size=6  marker2_edge_color=[0.85098 0.32549 0.0980392]  marker2_face_color=[0.85098 0.32549 0.0980392]  line3_style=Solid line (-)  line3_width=0.5  line3_color=[0.929412 0.694118 0.12549]  marker3=None  marker3_size=6  marker3_edge_color=[0.929412 0.694118 0.12549]  marker3_face_color=[0.929412 0.694118 0.12549]  line4_style=Solid line (-)  line4_width=0.5  line4_color=[0.494118 0.184314 0.556863]  marker4=None  marker4_size=6  marker4_edge_color=[0.494118 0.184314 0.556863]  marker4_face_color=[0.494118 0.184314 0.556863]  line5_style=Solid line (-)  line5_width=0.5  line5_color=[0.466667 0.67451 0.188235]  marker5=None  marker5_size=6  marker5_edge_color=[0.466667 0.67451 0.188235]  marker5_face_color=[0.466667 0.67451 0.188235]
      settings: SourceProductName=QUARC Targets
  Ranging Sensor Simulation : quarc_library/Devices/Third-Party/Sensors/Ranging Sensor Simulation  sensor_type=RPLIDAR A2  uri_source=External input port  uri=tcpip://localhost:18966  sample_time=qc_get_step_size * ceil(1/15 / qc_get_step_size)  show_in_use=off  variable_size=off  active=on
      settings: SourceProductName=QUARC Targets
  Reshape : Reshape  Commented=on  OutputDimensionality=Customize  OutputDimensions=[64,64]
  Reshape1 : Reshape  Commented=on  OutputDimensionality=Customize  OutputDimensions=[64,64]
  Slow to 5Hz : RateTransition  OutPortSampleTime=qc_get_step_size*ceil(1/15 / qc_get_step_size)
  Slow to 5Hz1 : RateTransition  OutPortSampleTime=qc_get_step_size*ceil(1/15 / qc_get_step_size)
  Slow to 5Hz2 : RateTransition  OutPortSampleTime=qc_get_step_size*ceil(1/15 / qc_get_step_size)
  Stream Server : quarc_library/Communications/Basic/Stream Server  Commented=on  uri_source=Specify via dialog (do not evaluate)  uri=tcpip://localhost:18966  send_buffer_size=8*4096*2  receive_buffer_size=1460  byte_order=little endian (Intel - LSB first)  optimization=Minimum latency  send_options=Send most recent data  receive_options=Do not receive data  default_value=[0]  sample_time=cameraStepSize  active=off  implementation=Use blocking I/O in a separate thread  send_fifo_size=1000  receive_fifo_size=1000  send_priority=0  receive_priority=0  send_dimensions=off  receive_dimensions=off  max_dimensions=-1  data_type=Inherited via back propagation  type_expr=BusObject
      settings: AttributesFormatString="\"tcpip://localhost:18966\""
  Terminator : Terminator  Commented=on
  Terminator1 : Terminator
  wires:
  Stream Server/1 -> Compare To Constant/1
  Compare To Constant/1 -> OR3/1
  Atomic Transition6/1 -> Stream Server/1
  Reshape/1 -> Matrix Concatenate/1
  Memory/1 -> Stream Server/2
  Reshape1/1 -> Matrix Concatenate/2
  OR3/1 -> Memory/1
  Stream Server/2 -> Compare To Constant1/1
  Matrix Concatenate/1 -> Atomic Transition6/1
  Compare To Constant1/1 -> OR3/2
  Stream Server/3 -> Terminator/1
  dist/1 -> Slow to 5Hz/1
  angles/1 -> Slow to 5Hz1/1
  Constant/1 -> Ranging Sensor Simulation/2
  Constant1/1 -> Ranging Sensor Simulation/5
  Constant2/1 -> Ranging Sensor Simulation/4
  Ranging Sensor Simulation/1 -> Terminator1/1
  Slow to 5Hz1/1 -> Polar Figure/2, Bias/1, Polar Figure1/2, Reshape1/1
  Slow to 5Hz/1 -> Gain/1, Polar Figure1/1, Reshape/1
  Gain/1 -> Polar Figure/1, Ranging Sensor Simulation/1
  Model Argument1/1 -> Slow to 5Hz2/1
  Slow to 5Hz2/1 -> Ranging Sensor Simulation/6
  Bias/1 -> Ranging Sensor Simulation/3

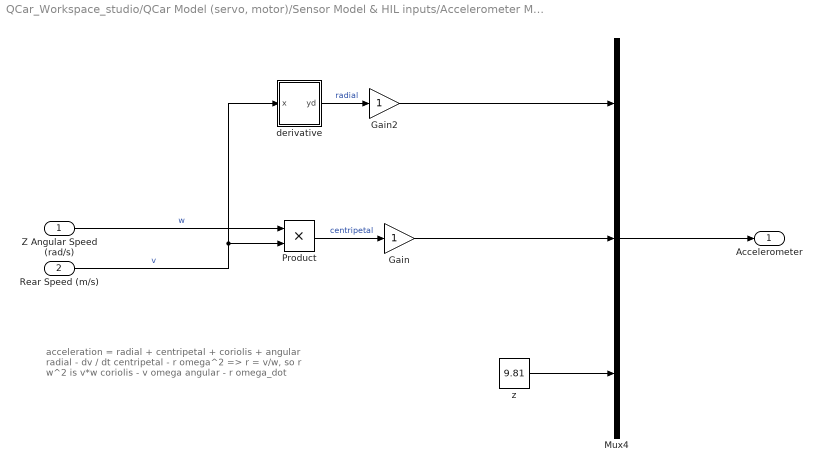
== system QCar_Workspace_studio/QCar Model (servo, motor)/Sensor Model & HIL inputs/Accelerometer Model1 ==
  note: acceleration = radial + centripetal + coriolis + angular
      |
      | radial		-	dv / dt
      | centripetal	-	r omega^2 => r = v/w, so r w^2 is v*w
      | coriolis		-	v omega
      | angular		-	r omega_dot
  Z Angular Speed (rad/s) : Inport
  Rear Speed (m/s) : Inport  Port=2
  Gain : Gain
  Gain2 : Gain
  Mux4 : Mux  Inputs=3
  Product : Product
  derivative : Subsystem
  z : Constant  Value=9.81
  Accelerometer : Outport
  wires:
  Z Angular Speed (rad/s)/1 -> Product/1  "w"
  derivative/1(yd) -> Gain2/1  "radial"
  Rear Speed (m/s)/1 -> Product/2, derivative/1(x)  "v"
  Product/1 -> Gain/1  "centripetal"
  Gain2/1 -> Mux4/1
  Gain/1 -> Mux4/2
  z/1 -> Mux4/3
  Mux4/1 -> Accelerometer/1

== system QCar_Workspace_studio/QCar Model (servo, motor)/Sensor Model & HIL inputs/Gyroscope Model ==
  Z Angular Speed (rad/s) : Inport
  Add2 : Sum
  Band-Limited White Noise : simulink/Sources/Band-Limited White Noise  Cov=[0.00001]  Ts=qc_get_step_size  seed=[23341]
  Mux4 : Mux  Inputs=2
  gyroscope : Constant  Value=[0 0 ]
  Gyroscope : Outport
  wires:
  Add2/1 -> Mux4/2
  gyroscope/1 -> Mux4/1
  Z Angular Speed (rad/s)/1 -> Add2/1
  Band-Limited White Noise/1 -> Add2/2
  Mux4/1 -> Gyroscope/1

== system QCar_Workspace_studio/QCar Model (servo, motor)/Sensor Model & HIL inputs/Accelerometer Model1/derivative ==
  x : Inport
  Constant : Constant
  Constant1 : Constant  Value=50
  Second-Order Low-Pass Filter : quarc_library/Continuous/Second-Order Low-Pass Filter  params_source=External (input ports)  input_width=1  input_zeta=1  input_init=0
  yd : Outport
  wires:
  x/1 -> Second-Order Low-Pass Filter/4, Second-Order Low-Pass Filter/1
  Constant1/1 -> Second-Order Low-Pass Filter/2
  Second-Order Low-Pass Filter/2 -> yd/1
  Constant/1 -> Second-Order Low-Pass Filter/3
